simulink model "Masse_MultirotorSimHinf"  (R2018b)
settings: Solver=VariableStepAuto  StartTime=0.0  StopTime=Simulation.T_END  MaxStep=Simulation.TS_MAX  RelTol=1e-3  EnableMultiTasking=on
PreLoadFcn:
  | % InitializeParameters;
undefined symbols (not defined in the file): Aero, armed, ctrl_state, INIT_PARAM_VECTOR, Initial, K_i, K_p, Motor, mpc_att_sp, mpc_ctrl_state, mpc_manual, mpc_pos_sp_triplet, mpc_vehicle_land_detected, mpc_vehicle_status, Simulation, SOF1, SOF2, Uav, Upsilon, v_att_sp, v_control_mode
libraries: simulink_extras x9, simulink x6, dspstat3 x1, Px4Library x1
(part 2 of 11)

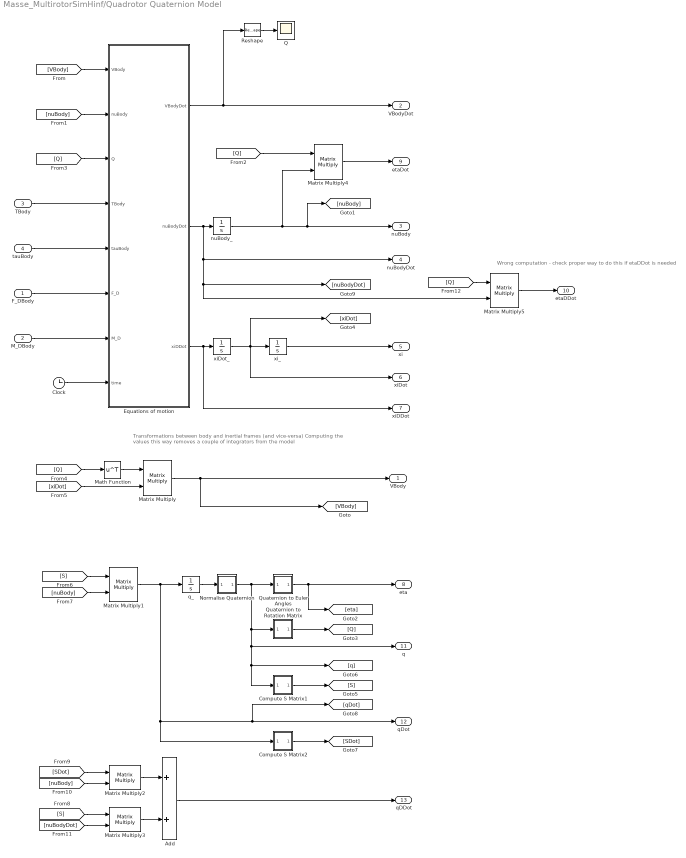
== system Masse_MultirotorSimHinf/Quadrotor Quaternion Model ==
  note: Wrong computation - check proper way to do this if etaDDot is needed
  note: Transformations between body and inertial frames (and vice-versa)
      | Computing the values this way removes a couple of integrators from the model
  F_DBody : Inport  Unit=N
  M_DBody : Inport  Port=2  Unit=N*m
  TBody : Inport  Port=3  Unit=N
  tauBody : Inport  Port=4  Unit=N*m
  Add : Sum
  Clock : Clock
  Compute S Matrix1 : Subsystem  AncestorBlock=QuaternionLibrary/Compute S Matrix
      mask help: Convert an orientation quaternion to an orthogonal transformation matrix
      mask Help:
      | Convert a quaternion
      | [q1 q2 q3 q4]
      | to the S matrix used to compute angular acceleration and velocity quaternion
      | qDot = S * nuBody
      | 
      | qDDot = SDot * nuBody + S * nuBodyDot
      mask Display: disp('S')
  Compute S Matrix2 : Subsystem  AncestorBlock=QuaternionLibrary/Compute S Matrix
      mask help: Convert an orientation quaternion to an orthogonal transformation matrix
      mask Help:
      | Convert a quaternion
      | [q1 q2 q3 q4]
      | to the S matrix used to compute angular acceleration and velocity quaternion
      | qDot = S * nuBody
      | 
      | qDDot = SDot * nuBody + S * nuBodyDot
      mask Display: disp('S')
  Equations of motion : MATLAB Function  TreatAsAtomicUnit=on
  Math Function : Math  Operator=transpose  SaturateOnIntegerOverflow=on
  Matrix Multiply{,1..5} (6 alike) : Product  Multiplication=Matrix(*)
  Normalise Quaternion : Subsystem  AncestorBlock=QuaternionLibrary/Normalise Quaternion
      mask help:
      | Normalise a quaternion
      |
      | Qhat = Q / |Q|
      mask Display: disp('Q/|Q|')
  Q : Scope
  Quaternion to Euler Angles : Subsystem  AncestorBlock=QuaternionLibrary/Quaternion to Euler Angles
      mask help: Convert an orientation quaternion to a vector of Euler angles
      mask Help:
      | Convert an orientation quaternion
      | [q1 q2 q3 q4]
      | where:
      | - q1 is the rotation in radians
      | - [q2 q3 q4] is the vector around which the rotation is performed)
      | to a vector of Euler angles
      | [roll, pitch, yaw]
      | Based on code from the PX4 firmware: https://github.com/PX4/Firmware
      mask Display: disp('Q2E')
  Quaternion to Rotation Matrix : Subsystem  AncestorBlock=QuaternionLibrary/Quaternion to Rotation Matrix
      mask help: Convert an orientation quaternion to an orthogonal transformation matrix
      mask Help:
      | Convert an orientation quaternion
      | [q1 q2 q3 q4]
      | where:
      | - q1 is the rotation in radians
      | - [q2 q3 q4] is the vector around which the rotation is performed)
      | to an orthogonal transformation matrix
      | Based on code from the PX4 firmware: https://github.com/PX4/Firmware
      mask Display: disp('Q2R')
  Reshape : Reshape  OutputDimensionality=Column vector (2-D)
  nuBody_ : Integrator  InitialCondition=Initial.NU_BODY
  q_ : Integrator  InitialCondition=Initial.Q
  xiDot_ : Integrator  InitialCondition=Initial.XI_DOT
  xi_ : Integrator  InitialCondition=Initial.XI
  VBody : Outport  Unit=m/s
  VBodyDot : Outport  Port=2  Unit=m/s^2
  nuBody : Outport  Port=3  Unit=rad/s
  nuBodyDot : Outport  Port=4  Unit=rad/s^2
  xi : Outport  Port=5  Unit=m
  xiDot : Outport  Port=6  Unit=m/s
  xiDDot : Outport  Port=7  Unit=m/s^2
  eta : Outport  Port=8  Unit=rad
  etaDot : Outport  Port=9  Unit=rad/s
  etaDDot : Outport  Port=10  Unit=rad/s^2
  q : Outport  Port=11
  qDot : Outport  Port=12
  qDDot : Outport  Port=13
  wires:
  Equations of motion/1(VBodyDot) -> Reshape/1, VBodyDot/1
  xi_/1 -> xi/1
  [nuBody] -> Equations of motion/2(nuBody)
  [VBody] -> Equations of motion/1(VBody)
  tauBody/1 -> Equations of motion/5(tauBody)
  TBody/1 -> Equations of motion/4(TBody)
  Equations of motion/3(xiDDot) -> xiDot_/1, xiDDot/1
  F_DBody/1 -> Equations of motion/6(F_D)
  Matrix Multiply/1 -> VBody/1, [VBody]
  M_DBody/1 -> Equations of motion/7(M_D)
  nuBody_/1 -> Matrix Multiply4/2, [nuBody], nuBody/1
  Equations of motion/2(nuBodyDot) -> nuBody_/1, nuBodyDot/1, Matrix Multiply5/2, [nuBodyDot]
  q_/1 -> Normalise Quaternion/1(quaternion)
  Quaternion to Euler Angles/1(euler) -> eta/1, [eta]
  Matrix Multiply4/1 -> etaDot/1
  Quaternion to Rotation Matrix/1(rotationMatrix) -> [Q]
  [Q] -> Equations of motion/3(Q)
  [Q] -> Math Function/1
  [xiDot] -> Matrix Multiply/2
  Math Function/1 -> Matrix Multiply/1
  [S] -> Matrix Multiply1/1
  [nuBody] -> Matrix Multiply1/2
  Compute S Matrix2/1(rotationMatrix) -> [SDot]
  [S] -> Matrix Multiply3/1
  Matrix Multiply1/1 -> qDot/1, [qDot], Compute S Matrix2/1(quaternion), q_/1
  [SDot] -> Matrix Multiply2/1
  [nuBody] -> Matrix Multiply2/2
  [nuBodyDot] -> Matrix Multiply3/2
  Matrix Multiply2/1 -> Add/1
  Matrix Multiply3/1 -> Add/2
  Normalise Quaternion/1(normalised) -> Quaternion to Euler Angles/1(quaternion), q/1, Compute S Matrix1/1(quaternion), [q], Quaternion to Rotation Matrix/1(quaternion)
  Compute S Matrix1/1(rotationMatrix) -> [S]
  [Q] -> Matrix Multiply4/1
  Add/1 -> qDDot/1
  [Q] -> Matrix Multiply5/1
  Matrix Multiply5/1 -> etaDDot/1
  Reshape/1 -> Q/1
  xiDot_/1 -> xi_/1, [xiDot], xiDot/1
  Clock/1 -> Equations of motion/8(time)

== system Masse_MultirotorSimHinf/Quaternion to Euler Angles ==
  quaternion : Inport
  MATLAB Function : MATLAB Function  TreatAsAtomicUnit=on
  euler : Outport
  wires:
  quaternion/1 -> MATLAB Function/1(quat)
  MATLAB Function/1(eul) -> euler/1

== system Masse_MultirotorSimHinf/Quaternion to Euler Angles1 ==
  quaternion : Inport
  MATLAB Function : MATLAB Function  TreatAsAtomicUnit=on
  euler : Outport
  wires:
  quaternion/1 -> MATLAB Function/1(quat)
  MATLAB Function/1(eul) -> euler/1

== system Masse_MultirotorSimHinf/SOF1 ==
  y1 : Inport
  Demux : Demux
  Demux1 : Demux  Outputs=2
  Demux2 : Demux  Outputs=2
  Ground : Ground
  Ground1 : Ground
  Manual Switch : ManualSwitch  CurrentSetting=0
  Mux : Mux
  Mux1 : Mux  Inputs=2
  Mux2 : Mux  Inputs=2
  Revert sign : Gain  Gain=-1
  Revert sign1 : Gain  Gain=-1
  SOF1 : Gain  Gain=SOF1  Multiplication=Matrix(K*u)
  SOF1_21-32 : Gain  Gain=-0.76671643026053
  SOF1_23-34 : Gain  Gain=-1.44072900590537
  Sum : Sum  Inputs=+|+
  Sum1 : Sum  Inputs=+|+
  u1 : Outport
  wires:
  Mux/1 -> Manual Switch/2
  Demux/4 -> Mux2/2  "x"
  Demux/3 -> Mux2/1  "y"
  Demux/2 -> Mux1/2  "xdot"
  Demux/1 -> Mux1/1  "ydot"
  Sum1/1 -> Mux/3
  Sum/1 -> Mux/2
  Demux1/1 -> Revert sign/1
  SOF1/1 -> Manual Switch/1
  Manual Switch/1 -> u1/1
  y1/1 -> SOF1/1, Demux/1
  Ground/1 -> Mux/4
  Ground1/1 -> Mux/1
  Demux2/1 -> Revert sign1/1
  SOF1_21-32/1 -> Demux1/1
  Mux1/1 -> SOF1_21-32/1
  Demux1/2 -> Sum1/1
  Mux2/1 -> SOF1_23-34/1
  SOF1_23-34/1 -> Demux2/1
  Demux2/2 -> Sum1/2
  Revert sign/1 -> Sum/1
  Revert sign1/1 -> Sum/2

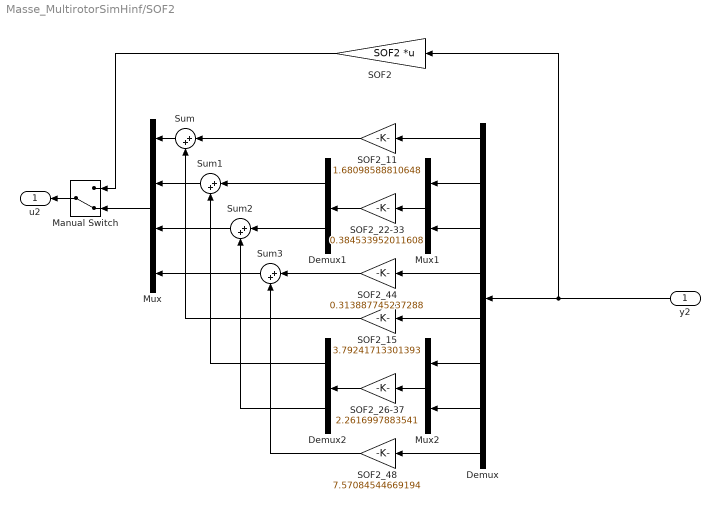
== system Masse_MultirotorSimHinf/SOF2 ==
  y2 : Inport
  Demux : Demux  Outputs=8
  Demux1 : Demux  Outputs=2
  Demux2 : Demux  Outputs=2
  Manual Switch : ManualSwitch  CurrentSetting=0
  Mux : Mux
  Mux1 : Mux  Inputs=2
  Mux2 : Mux  Inputs=2
  SOF2 : Gain  Gain=SOF2  Multiplication=Matrix(K*u)
  SOF2_11 : Gain  Gain=1.68098588810648
  SOF2_15 : Gain  Gain=3.79241713301393
  SOF2_22-33 : Gain  Gain=0.384533952011608
  SOF2_26-37 : Gain  Gain=2.2616997883541
  SOF2_44 : Gain  Gain=0.313887745237288
  SOF2_48 : Gain  Gain=7.57084544669194
  Sum{,1..3} (4 alike) : Sum  Inputs=|++
  u2 : Outport
  wires:
  y2/1 -> SOF2/1, Demux/1
  Manual Switch/1 -> u2/1
  SOF2/1 -> Manual Switch/1
  SOF2_11/1 -> Sum/1
  Demux1/1 -> Sum1/1
  Demux1/2 -> Sum2/1
  SOF2_44/1 -> Sum3/1
  SOF2_15/1 -> Sum/2
  Demux2/1 -> Sum1/2
  Demux2/2 -> Sum2/2
  SOF2_48/1 -> Sum3/2
  Demux/1 -> SOF2_11/1
  Demux/2 -> Mux1/1
  Demux/3 -> Mux1/2
  Demux/4 -> SOF2_44/1
  Demux/5 -> SOF2_15/1
  Demux/6 -> Mux2/1
  Demux/7 -> Mux2/2
  Demux/8 -> SOF2_48/1
  Mux/1 -> Manual Switch/2
  Sum3/1 -> Mux/4
  Sum2/1 -> Mux/3
  Sum1/1 -> Mux/2
  Sum/1 -> Mux/1
  Mux2/1 -> SOF2_26-37/1
  SOF2_26-37/1 -> Demux2/1
  SOF2_22-33/1 -> Demux1/1
  Mux1/1 -> SOF2_22-33/1

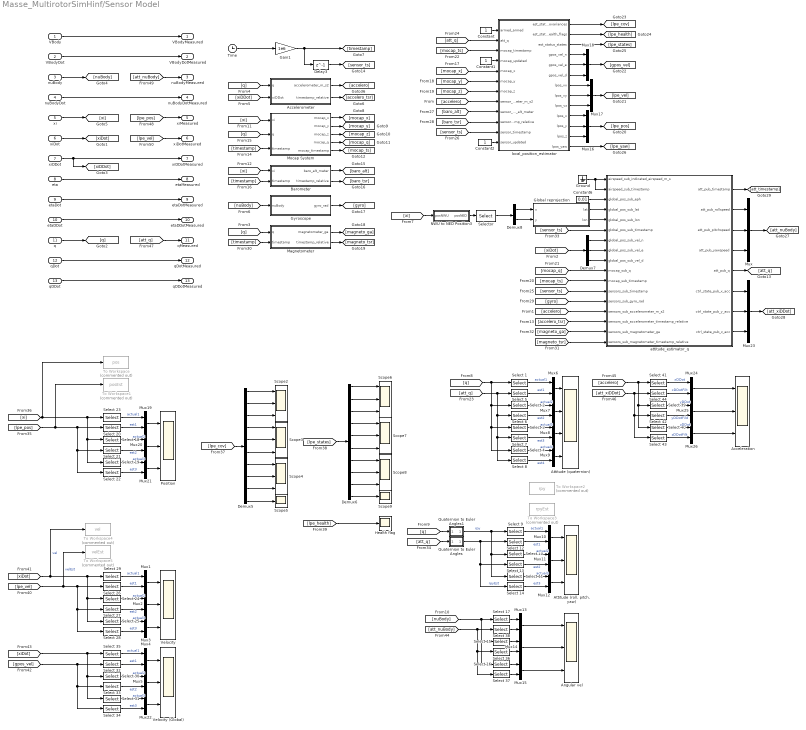
== system Masse_MultirotorSimHinf/Sensor Model ==
  VBody : Inport  Unit=m/s  PortDimensions=3
  VBodyDot : Inport  Port=2  Unit=m/s^2  PortDimensions=3
  nuBody : Inport  Port=3  Unit=rad/s  PortDimensions=3
  nuBodyDot : Inport  Port=4  Unit=rad/s^2  PortDimensions=3
  xi : Inport  Port=5  Unit=m  PortDimensions=3
  xiDot : Inport  Port=6  Unit=m/s  PortDimensions=3
  xiDDot : Inport  Port=7  Unit=m/s^2  PortDimensions=3
  eta : Inport  Port=8  Unit=rad  PortDimensions=3
  etaDot : Inport  Port=9  Unit=rad/s  PortDimensions=3
  etaDDot : Inport  Port=10  Unit=rad/s^2  PortDimensions=3
  q : Inport  Port=11  PortDimensions=4
  qDot : Inport  Port=12  PortDimensions=4
  qDDot : Inport  Port=13  PortDimensions=4
  Acceleration : Scope  NumInputPorts=3
  Accelerometer : Subsystem
  Angular vel : Scope  NumInputPorts=3
  Attitude (quaternion) : Scope  NumInputPorts=4
  "Attitude (roll, pitch, yaw)" : Scope  NumInputPorts=3
  Barometer : Subsystem
  Constant : Constant
  Constant1 : Constant
  Constant2 : Constant
  Constant6 : Constant  Value=0.01
  Delay3 : Delay  DelayLength=1  SampleTime=1/400
  Demux5 : Demux  Outputs=10
  Demux6 : Demux  Outputs=10
  Demux7 : Demux  Outputs=3
  Demux8 : Demux  Outputs=2
  Gain1 : Gain  Gain=1e6
  Global reprojection : Subsystem  AncestorBlock=Px4Library/Global reprojection  mask{LAT0=-36.865577, LON0=174.772065}
      mask prompts: LAT0 "Latitude at [x,y] = [0,0]"; LON0 "Longitude at [x,y] = [0,0]"
      mask Display:
      | disp('REPROJECT')
      | port_label('input', 1, sprintf('x'))
      | port_label('input', 2, sprintf('y'))
      | port_label('output', 1, sprintf('lat'))
      | port_label('output', 2, sprintf('lon'))
  Ground : Ground
  Gyroscope : Subsystem
  Health flag : Scope
  Magnetometer : Subsystem
  Mocap System : Subsystem
  Mux{,16..18,23} (5 alike) : Mux  Inputs=3
  Mux{1..15,19..22,24..26} (22 alike) : Mux  Inputs=2
  NWU to NED Position3 : Subsystem  AncestorBlock=Px4Library/NWU to NED Position  mask(Coordinate transform){}
      mask help:
      | Convert a 3x1 vector or 4x1 quaternion from a North West Up to a North East Down coordinate system.
      |
      | The appropriate coordinate transform is automatically selected based on the input size.
  Position : Scope  NumInputPorts=3
  Quaternion to Euler Angles : Subsystem  AncestorBlock=QuaternionLibrary/Quaternion to Euler Angles
      mask help: Convert an orientation quaternion to a vector of Euler angles
      mask Help:
      | Convert an orientation quaternion
      | [q1 q2 q3 q4]
      | where:
      | - q1 is the rotation in radians
      | - [q2 q3 q4] is the vector around which the rotation is performed)
      | to a vector of Euler angles
      | [roll, pitch, yaw]
      | Based on code from the PX4 firmware: https://github.com/PX4/Firmware
      mask Display: disp('Q2E')
  Quaternion to Euler Angles1 : Subsystem  AncestorBlock=QuaternionLibrary/Quaternion to Euler Angles
      mask help: Convert an orientation quaternion to a vector of Euler angles
      mask Help:
      | Convert an orientation quaternion
      | [q1 q2 q3 q4]
      | where:
      | - q1 is the rotation in radians
      | - [q2 q3 q4] is the vector around which the rotation is performed)
      | to a vector of Euler angles
      | [roll, pitch, yaw]
      | Based on code from the PX4 firmware: https://github.com/PX4/Firmware
      mask Display: disp('Q2E')
  Scope{2..4,6..8} (6 alike) : Scope  NumInputPorts=3
  Scope5 : Scope
  Scope9 : Scope
  Select 1 : Selector  InputPortWidth=4  IndexOptions=Index vector (dialog)  Indices=1  OutputSizes=1
  Select {10,13,15,18,21,24,27,30,33,36,39,42} (12 alike) : Selector  InputPortWidth=3  IndexOptions=Index vector (dialog)  Indices=2  OutputSizes=1
  Select {11,14,16,19,22,25,28,31,34,37,40,43} (12 alike) : Selector  InputPortWidth=3  IndexOptions=Index vector (dialog)  Indices=3  OutputSizes=1
  Select {9,12,17,20,23,26,29,32,35,38,41,44} (12 alike) : Selector  InputPortWidth=3  IndexOptions=Index vector (dialog)  Indices=1  OutputSizes=1
  Select 2 : Selector  InputPortWidth=4  IndexOptions=Index vector (dialog)  Indices=2  OutputSizes=1
  Select 3 : Selector  InputPortWidth=4  IndexOptions=Index vector (dialog)  Indices=3  OutputSizes=1
  Select 4 : Selector  InputPortWidth=4  IndexOptions=Index vector (dialog)  Indices=4  OutputSizes=1
  Select 5 : Selector  InputPortWidth=4  IndexOptions=Index vector (dialog)  Indices=1  OutputSizes=1
  Select 6 : Selector  InputPortWidth=4  IndexOptions=Index vector (dialog)  Indices=2  OutputSizes=1
  Select 7 : Selector  InputPortWidth=4  IndexOptions=Index vector (dialog)  Indices=3  OutputSizes=1
  Select 8 : Selector  InputPortWidth=4  IndexOptions=Index vector (dialog)  Indices=4  OutputSizes=1
  Selector : Selector  InputPortWidth=3  IndexOptions=Index vector (dialog)  Indices=[1 2]  OutputSizes=1
  Time : Clock
  To Workspace : ToWorkspace  Commented=on  VariableName=pos  SaveFormat=Structure With Time  SampleTime=-1
  To Workspace1 : ToWorkspace  Commented=on  VariableName=posEst  SaveFormat=Structure With Time  SampleTime=-1
  To Workspace2 : ToWorkspace  Commented=on  VariableName=rpy  SaveFormat=Structure With Time  SampleTime=-1
  To Workspace3 : ToWorkspace  Commented=on  VariableName=rpyEst  SaveFormat=Structure With Time  SampleTime=-1
  To Workspace4 : ToWorkspace  Commented=on  VariableName=vel  SaveFormat=Structure With Time  SampleTime=-1
  To Workspace5 : ToWorkspace  Commented=on  VariableName=velEst  SaveFormat=Structure With Time  SampleTime=-1
  Velocity : Scope  NumInputPorts=3
  Velocity (Global) : Scope  NumInputPorts=3
  attitude_estimator_q : Subsystem  AncestorBlock=Px4Library/attitude_estimator_q  mask(PX4 LPE (local position estimator): local_position_estimator){Q_SAMPLING_PERIOD=1/250, INIT_Q=[0.99812 -1.4569e-22   -0.061217 -8.9353e-24], ATT_W_ACC=0.2, ATT_W_MAG=0.1, ATT_W_EXT_HDG=0.1, ATT_W_GYRO_BIAS=0.1, ATT_MAG_DECL=0, ATT_MAG_DECL_A=1, ATT_EXT_HDG_M=2, ATT_ACC_COMP=1, ATT_BIAS_MAX=0.05, FW_ARSP_MODE=0}
      mask prompts: Q_SAMPLING_PERIOD "Sampling period (s)"; INIT_Q "INIT_Q - Initial UAV orientation - set to 0 to let controller decide (bugged) (-)"; ATT_W_ACC "ATT_W_ACC - Complimentary filter accelerometer weight (-)"; ATT_W_MAG "ATT_W_MAG - Complimentary filter magnetometer weight (-)"; ATT_W_EXT_HDG "ATT_W_EXT_HDG - Complimentary filter external heading weight (-)"; ATT_W_GYRO_BIAS "ATT_W_GYRO_BIAS - Complimentary filter gyroscope bias weight (-)"; ATT_MAG_DECL "ATT_MAG_DECL - Magnetic declination. Not used when GPS available (deg)"; ATT_MAG_DECL_A "ATT_MAG_DECL_A - Automatic GPS based declination compensation (-)"; ATT_EXT_HDG_M "ATT_EXT_HDG_M - External heading usage mode (from Motion capture/Vision) (-), 0 None 1 Vision 2 Motion Capture"; ATT_ACC_COMP "ATT_ACC_COMP - Acceleration compensation based on GPS velocity. (-)"; ATT_BIAS_MAX "ATT_BIAS_MAX - Gyro bias limit (rad/s)"; FW_ARSP_MODE "FW_ARSP_MODE - Method used to publish the airspeed (-), 0 Measured airspeed 1 Vehicle ground speed 2 Airspeed invalid"
      mask TypeOptions ATT_EXT_HDG_M: 0 | 1 | 2
      mask TypeOptions FW_ARSP_MODE: 0 | 1 | 2
  local_position_estimator : Subsystem  AncestorBlock=Px4Library/local_position_estimator  mask(PX4 LPE (local position estimator): local_position_estimator){LPE_SAMPLING_PERIOD=0.01, LPE_ACC_XY=0.012, LPE_ACC_Z=0.02, LPE_BAR_Z=3, LPE_EPH_MAX=3, LPE_EPV_MAX=5, LPE_FAKE_ORIGIN=0, LPE_FGYRO_HP=0.001, LPE_FLW_OFF_Z=0, LPE_FLW_QMIN=150, LPE_FLW_R=7, LPE_FLW_RR=7, LPE_FLW_SCALE=1.3, LPE_GPS_DELAY=0.29, LPE_GPS_VXY=0.25, LPE_GPS_VZ=0.25, LPE_GPS_XY=1, LPE_GPS_Z=3, LPE_LAND_VXY=0.05, LPE_LAND_Z=0.03, LPE_LAT=40.43, LPE_LDR_OFF_Z=0, LPE_LDR_Z=0.03, LPE_LON=-86.929, LPE_PN_B=0.001, LPE_PN_P=0.1, LPE_PN_T=0.001, LPE_PN_V=0.1, LPE_SNR_OFF_Z=0, LPE_SNR_Z=0.05, LPE_T_MAX_GRADE=1, LPE_VIC_P=0.001, LPE_VIS_DELAY=0.1, LPE_VIS_XY=0.1, LPE_VIS_Z=0.5, LPE_VXY_PUB=0.3, LPE_X_LP=5, LPE_Z_PUB=1, LPE_FUSION=193, Barometer=on, GPS=off, LIDAR=off, Flow=off, Sonar=off, Vision=off, Mocap=on, Land=on}
      mask prompts: LPE_SAMPLING_PERIOD "Sampling period (s)"; LPE_ACC_XY "LPE_ACC_XY - Accelerometer xy noise density (m/s^2/sqrt(Hz))"; LPE_ACC_Z "LPE_ACC_Z - Accelerometer z noise density (m/s^2/sqrt(Hz))"; LPE_BAR_Z "LPE_BAR_Z - Barometric presssure altitude z standard deviation. (m)"; LPE_EPH_MAX "LPE_EPH_MAX - Max EPH allowed for GPS initialization (m)"; LPE_EPV_MAX "LPE_EPV_MAX - Max EPV allowed for GPS initialization (m)"; LPE_FAKE_ORIGIN "LPE_FAKE_ORIGIN - Enable publishing of a fake global position (e.g for AUTO missions using Optical Flow) (-)"; LPE_FGYRO_HP "LPE_FGYRO_HP - Flow gyro high pass filter cut off frequency (Hz)"; LPE_FLW_OFF_Z "LPE_FLW_OFF_Z - Optical flow z offset from center (m)"; LPE_FLW_QMIN "LPE_FLW_QMIN - Optical flow minimum quality threshold (-)"; LPE_FLW_R "LPE_FLW_R - Optical flow rotation (roll/pitch) noise gain (m/s / (rad))"; LPE_FLW_RR "LPE_FLW_RR - Optical flow angular velocity noise gain (m/s / (rad/s))"; LPE_FLW_SCALE "LPE_FLW_SCALE - Optical flow scale (m)"; LPE_GPS_DELAY "LPE_GPS_DELAY - GPS delay compensaton (sec)"; LPE_GPS_VXY "LPE_GPS_VXY - GPS xy velocity standard deviation. (m/s)"; LPE_GPS_VZ "LPE_GPS_VZ - GPS z velocity standard deviation. (m/s)"; LPE_GPS_XY "LPE_GPS_XY - Minimum GPS xy standard deviation, uses reported EPH if greater. (m)"; LPE_GPS_Z "LPE_GPS_Z - Minimum GPS z standard deviation, uses reported EPV if greater. (m)"; LPE_LAND_VXY "LPE_LAND_VXY - Land detector xy velocity standard deviation (m/s)"; LPE_LAND_Z "LPE_LAND_Z - Land detector z standard deviation (m)"; LPE_LAT "LPE_LAT - Local origin latitude for nav w/o GPS (deg)"; LPE_LDR_OFF_Z "LPE_LDR_OFF_Z - Lidar z offset from center of vehicle +down (m)"; LPE_LDR_Z "LPE_LDR_Z - Lidar z standard deviation. (m)"; LPE_LON "LPE_LON - Local origin longitude for nav w/o GPS (deg)"; LPE_PN_B "LPE_PN_B - Accel bias propagation noise density ((m/s^2)/s/sqrt(Hz))"; LPE_PN_P "LPE_PN_P - Position propagation noise density (m/s/sqrt(Hz))"; LPE_PN_T "LPE_PN_T - Terrain random walk noise density, hilly/outdoor (0.1), flat/Indoor (0.001) ((m/s)/(sqrt(hz)))"; LPE_PN_V "LPE_PN_V - Velocity propagation noise density ((m/s)/s/sqrt(Hz))"; LPE_SNR_OFF_Z "LPE_SNR_OFF_Z - Sonar z offset from center of vehicle +down (m)"; LPE_SNR_Z "LPE_SNR_Z - Sonar z standard deviation. (m)"; LPE_T_MAX_GRADE "LPE_T_MAX_GRADE - Terrain maximum percent grade, hilly/outdoor (100 = 45 deg), flat/Indoor (0 = 0 deg) (%)"; LPE_VIC_P "LPE_VIC_P - Vicon position standard deviation. (m)"; LPE_VIS_DELAY "LPE_VIS_DELAY - Vision delay compensaton. (sec)"; LPE_VIS_XY "LPE_VIS_XY - Vision xy standard deviation. (m)"; LPE_VIS_Z "LPE_VIS_Z - Vision z standard deviation. (m)"; LPE_VXY_PUB "LPE_VXY_PUB - Required velocity xy standard deviation to publish position (m/s)"; LPE_X_LP "LPE_X_LP - Cut frequency for state publication (Hz)"; LPE_Z_PUB "LPE_Z_PUB - Required z standard deviation to publish altitude/ terrain (m)"; LPE_FUSION "LPE_FUSION - Integer bitmask controlling data fusion (-)"; Barometer "Use Barometer"; GPS "Use GPS"; LIDAR "Use LIDAR"; Flow "Use Flow"; Sonar "Use Sonar"; Vision "Use Vision"; Mocap "Use Mocap"; Land "Use Land"
      mask Callback Barometer:
      | status = get_param( gcb, 'Barometer' );
      | if strcmp( status, 'on' )
      | 	lpe = bitor( uint8(str2num(get_param( gcb, 'LPE_FUSION' ))), uint8(2^0) );
      | 	set_param( gcb, 'LPE_FUSION', num2str(lpe) );
      | else
      | 	lpe = bitand( uint8(str2num(get_param( gcb, 'LPE_FUSION' ))), bitcmp(uint8(2^0), 'uint8' ));
      | 	set_param( gcb, 'LPE_FUSION', num2str(lpe) );
      | end
      mask Callback GPS:
      | status = get_param( gcb, 'GPS' );
      | if strcmp( status, 'on' )
      | 	lpe = bitor( uint8(str2num(get_param( gcb, 'LPE_FUSION' ))), uint8(2^1) );
      | 	set_param( gcb, 'LPE_FUSION', num2str(lpe) );
      | else
      | 	lpe = bitand( uint8(str2num(get_param( gcb, 'LPE_FUSION' ))), bitcmp(uint8(2^1), 'uint8' ));
      | 	set_param( gcb, 'LPE_FUSION', num2str(lpe) );
      | end
      mask Callback LIDAR:
      | status = get_param( gcb, 'LIDAR' );
      | if strcmp( status, 'on' )
      | 	lpe = bitor( uint8(str2num(get_param( gcb, 'LPE_FUSION' ))), uint8(2^2) );
      | 	set_param( gcb, 'LPE_FUSION', num2str(lpe) );
      | else
      | 	lpe = bitand( uint8(str2num(get_param( gcb, 'LPE_FUSION' ))), bitcmp(uint8(2^2), 'uint8' ));
      | 	set_param( gcb, 'LPE_FUSION', num2str(lpe) );
      | end
      mask Callback Flow:
      | status = get_param( gcb, 'Flow' );
      | if strcmp( status, 'on' )
      | 	lpe = bitor( uint8(str2num(get_param( gcb, 'LPE_FUSION' ))), uint8(2^3) );
      | 	set_param( gcb, 'LPE_FUSION', num2str(lpe) );
      | else
      | 	lpe = bitand( uint8(str2num(get_param( gcb, 'LPE_FUSION' ))), bitcmp(uint8(2^3), 'uint8' ));
      | 	set_param( gcb, 'LPE_FUSION', num2str(lpe) );
      | end
      mask Callback Sonar:
      | status = get_param( gcb, 'Sonar' );
      | if strcmp( status, 'on' )
      | 	lpe = bitor( uint8(str2num(get_param( gcb, 'LPE_FUSION' ))), uint8(2^4) );
      | 	set_param( gcb, 'LPE_FUSION', num2str(lpe) );
      | else
      | 	lpe = bitand( uint8(str2num(get_param( gcb, 'LPE_FUSION' ))), bitcmp(uint8(2^4), 'uint8' ));
      | 	set_param( gcb, 'LPE_FUSION', num2str(lpe) );
      | end
      mask Callback Vision:
      | status = get_param( gcb, 'Vision' );
      | if strcmp( status, 'on' )
      | 	lpe = bitor( uint8(str2num(get_param( gcb, 'LPE_FUSION' ))), uint8(2^5) );
      | 	set_param( gcb, 'LPE_FUSION', num2str(lpe) );
      | else
      | 	lpe = bitand( uint8(str2num(get_param( gcb, 'LPE_FUSION' ))), bitcmp(uint8(2^5), 'uint8' ));
      | 	set_param( gcb, 'LPE_FUSION', num2str(lpe) );
      | end
      mask Callback Mocap:
      | status = get_param( gcb, 'Mocap' );
      | if strcmp( status, 'on' )
      | 	lpe = bitor( uint8(str2num(get_param( gcb, 'LPE_FUSION' ))), uint8(2^6) );
      | 	set_param( gcb, 'LPE_FUSION', num2str(lpe) );
      | else
      | 	lpe = bitand( uint8(str2num(get_param( gcb, 'LPE_FUSION' ))), bitcmp(uint8(2^6), 'uint8' ));
      | 	set_param( gcb, 'LPE_FUSION', num2str(lpe) );
      | end
      mask Callback Land:
      | status = get_param( gcb, 'Land' );
      | if strcmp( status, 'on' )
      | 	lpe = bitor( uint8(str2num(get_param( gcb, 'LPE_FUSION' ))), uint8(2^7) );
      | 	set_param( gcb, 'LPE_FUSION', num2str(lpe) );
      | else
      | 	lpe = bitand( uint8(str2num(get_param( gcb, 'LPE_FUSION' ))), bitcmp(uint8(2^7), 'uint8' ));
      | 	set_param( gcb, 'LPE_FUSION', num2str(lpe) );
      | end
  VBodyMeasured : Outport  Unit=m/s
  VBodyDotMeasured : Outport  Port=2  Unit=m/s^2
  nuBodyMeasured : Outport  Port=3  Unit=rad/s
  nuBodyDotMeasured : Outport  Port=4  Unit=rad/s^2
  xiMeasured : Outport  Port=5  Unit=m
  xiDotMeasured : Outport  Port=6  Unit=m/s
  xiDDotMeasured : Outport  Port=7  Unit=m/s^2
  etaMeasured : Outport  Port=8  Unit=rad
  etaDotMeasured : Outport  Port=9  Unit=rad/s
  etaDDotMeasured : Outport  Port=10  Unit=rad/s^2
  qMeasured : Outport  Port=11
  qDotMeasured : Outport  Port=12
  qDDotMeasured : Outport  Port=13
  wires:
  xiDot/1 -> [xiDot]
  xi/1 -> [xi]
  nuBodyDot/1 -> nuBodyDotMeasured/1
  nuBody/1 -> [nuBody]
  VBodyDot/1 -> VBodyDotMeasured/1
  VBody/1 -> VBodyMeasured/1
  eta/1 -> etaMeasured/1
  etaDot/1 -> etaDotMeasured/1
  etaDDot/1 -> etaDDotMeasured/1
  q/1 -> [q]
  qDot/1 -> qDotMeasured/1
  qDDot/1 -> qDDotMeasured/1
  [att_q] -> local_position_estimator/2(att_q)
  [mocap_x] -> local_position_estimator/5(mocap_x)
  [mocap_z] -> local_position_estimator/7(mocap_z)
  local_position_estimator/10(lpos_x) -> Mux16/1
  local_position_estimator/11(lpos_y) -> Mux16/2
  local_position_estimator/12(lpos_z) -> Mux16/3
  Demux5/2 -> Scope2/2
  Demux5/1 -> Scope2/1
  Demux5/3 -> Scope2/3
  Demux5/4 -> Scope3/1
  Demux5/5 -> Scope3/2
  Demux5/6 -> Scope3/3
  Demux5/7 -> Scope4/1
  Demux5/8 -> Scope4/2
  Demux5/9 -> Scope4/3
  Demux5/10 -> Scope5/1
  [lpe_states] -> Demux6/1
  Demux6/2 -> Scope6/2
  Demux6/1 -> Scope6/1
  Demux6/3 -> Scope6/3
  Demux6/4 -> Scope7/1
  Demux6/5 -> Scope7/2
  Demux6/6 -> Scope7/3
  Demux6/7 -> Scope8/1
  Demux6/8 -> Scope8/2
  Demux6/9 -> Scope8/3
  Demux6/10 -> Scope9/1
  Constant1/1 -> local_position_estimator/4(mocap_updated)
  [lpe_health] -> Health flag/1
  Constant/1 -> local_position_estimator/1(armed_armed)
  [mocap_ts] -> local_position_estimator/3(mocap_timestamp)
  [xiDot] -> Demux7/1
  Time/1 -> Gain1/1
  [accelero_tsr] -> attitude_estimator_q/15(sensors_sub_accelerometer_timestamp_relative)
  Global reprojection/1(lat) -> attitude_estimator_q/4(global_pos_sub_lat)
  Global reprojection/2(lon) -> attitude_estimator_q/5(global_pos_sub_lon)
  [xi] -> NWU to NED Position3/1(posNWU)
  NWU to NED Position3/1(posNED) -> Selector/1
  Selector/1 -> Demux8/1
  Demux8/1 -> Global reprojection/1(x)
  Demux8/2 -> Global reprojection/2(y)
  [att_q] -> Select 8/1, Select 7/1, Select 6/1, Select 5/1
  [q] -> Select 2/1, Select 3/1, Select 4/1, Select 1/1
  Mux6/1 -> Attitude (quaternion)/1
  Mux7/1 -> Attitude (quaternion)/2
  Mux8/1 -> Attitude (quaternion)/3
  Mux9/1 -> Attitude (quaternion)/4
  Select 4/1 -> Mux9/1  "actual4"
  Select 8/1 -> Mux9/2  "est4"
  Select 3/1 -> Mux8/1  "actual3"
  Select 7/1 -> Mux8/2  "est3"
  Select 6/1 -> Mux7/2  "est2"
  Select 2/1 -> Mux7/1  "actual2"
  Select 5/1 -> Mux6/2  "est1"
  Select 1/1 -> Mux6/1  "actual1"
  Constant6/1 -> attitude_estimator_q/3(global_pos_sub_eph)
  [q] -> Magnetometer/1(q)
  Mux10/1 -> "Attitude (roll, pitch, yaw)"/1
  Mux11/1 -> "Attitude (roll, pitch, yaw)"/2
  Mux12/1 -> "Attitude (roll, pitch, yaw)"/3
  Select 11/1 -> Mux12/1  "actual3"
  Select 14/1 -> Mux12/2  "est3"
  Select 13/1 -> Mux11/2  "est2"
  Select 10/1 -> Mux11/1  "actual2"
  Select 12/1 -> Mux10/2  "est1"
  Select 9/1 -> Mux10/1  "actual1"
  [q] -> Quaternion to Euler Angles1/1(quaternion)
  Quaternion to Euler Angles1/1(euler) -> Select 11/1, Select 10/1, Select 9/1  "rpy"
  Quaternion to Euler Angles/1(euler) -> Select 14/1, Select 13/1, Select 12/1  "rpyEst"
  Mux13/1 -> Angular vel/1
  Mux14/1 -> Angular vel/2
  Mux15/1 -> Angular vel/3
  Select 17/1 -> Mux13/1
  Select 15/1 -> Mux14/1
  Select 16/1 -> Mux15/1
  [nuBody] -> Select 17/1, Select 16/1, Select 15/1
  Demux7/2 -> attitude_estimator_q/8(global_pos_sub_vel_e)
  [accelero] -> attitude_estimator_q/14(sensors_sub_accelerometer_m_s2)
  [sensor_ts] -> attitude_estimator_q/12(sensors_sub_timestamp)
  [magneto_ga] -> attitude_estimator_q/16(sensors_sub_magnetometer_ga)
  [nuBody] -> Gyroscope/1(nuBody)
  [gyro] -> attitude_estimator_q/13(sensors_sub_gyro_rad)
  [q] -> Accelerometer/1(q)
  [xiDDot] -> Accelerometer/2(xiDDot)
  Accelerometer/1(accelerometer_m_s2) -> [accelero]
  Accelerometer/2(timestamp_relative) -> [accelero_tsr]
  [mocap_q] -> attitude_estimator_q/10(mocap_sub_q)
  [mocap_ts] -> attitude_estimator_q/11(mocap_sub_timestamp)
  Gain1/1 -> Delay3/1, [timestamp]
  [timestamp] -> Mocap System/3(timestamp)
  [q] -> Mocap System/2(q)
  [xi] -> Mocap System/1(xi)
  Constant2/1 -> local_position_estimator/12(sensor_updated)
  [baro_alt] -> local_position_estimator/9(sensor_baro_alt_meter)
  [baro_tsr] -> local_position_estimator/10(sensor_baro_timestamp_relative)
  Mocap System/1(mocap_x) -> [mocap_x]
  Mocap System/2(mocap_y) -> [mocap_y]
  Mocap System/3(mocap_z) -> [mocap_z]
  [mocap_y] -> local_position_estimator/6(mocap_y)
  Mocap System/4(mocap_q) -> [mocap_q]
  Mocap System/5(mocap_timestamp) -> [mocap_ts]
  attitude_estimator_q/5(att_pub_q) -> [att_q]
  Delay3/1 -> [sensor_ts]
  [sensor_ts] -> local_position_estimator/11(sensor_timestamp)
  [xi] -> Barometer/1(xi)
  [timestamp] -> Barometer/2(timestamp)
  Barometer/1(baro_alt_meter) -> [baro_alt]
  Barometer/2(timestamp_relative) -> [baro_tsr]
  Gyroscope/1(gyro_rad) -> [gyro]
  [timestamp] -> Magnetometer/2(timestamp)
  Magnetometer/2(timestamp_relative) -> [magneto_tsr]
  Magnetometer/1(magnetometer_ga) -> [magneto_ga]
  [magneto_tsr] -> attitude_estimator_q/17(sensors_sub_magnetometer_timestamp_relative)
  Demux7/1 -> attitude_estimator_q/7(global_pos_sub_vel_n)
  Demux7/3 -> attitude_estimator_q/9(global_pos_sub_vel_d)
  [sensor_ts] -> attitude_estimator_q/6(global_pos_sub_timestamp)
  Mux16/1 -> [lpe_pos]
  local_position_estimator/7(lpos_vx) -> Mux17/1
  local_position_estimator/8(lpos_vy) -> Mux17/2
  local_position_estimator/9(lpos_vz) -> Mux17/3
  Mux17/1 -> [lpe_vel]
  local_position_estimator/4(gpos_vel_n) -> Mux18/1
  local_position_estimator/5(gpos_vel_e) -> Mux18/2
  local_position_estimator/6(gpos_vel_d) -> Mux18/3
  Mux18/1 -> [gpos_vel]
  local_position_estimator/1(est_status_covariances) -> [lpe_cov]
  local_position_estimator/2(est_status_health_flags) -> [lpe_health]
  local_position_estimator/3(est_status_states) -> [lpe_states]
  [att_q] -> Quaternion to Euler Angles/1(quaternion)
  Mux19/1 -> Position/1
  Mux20/1 -> Position/2
  Mux21/1 -> Position/3
  Select 19/1 -> Mux21/1  "actual3"
  Select 22/1 -> Mux21/2  "est3"
  Select 21/1 -> Mux20/2  "est2"
  Select 18/1 -> Mux20/1  "actual2"
  Select 20/1 -> Mux19/2  "est1"
  Select 23/1 -> Mux19/1  "actual1"
  [lpe_pos] -> To Workspace1/1, Select 20/1, Select 21/1, Select 22/1
  [lpe_cov] -> Demux5/1
  [xi] -> Select 23/1, Select 18/1, Select 19/1, To Workspace/1
  Mux1/1 -> Velocity/1
  Mux2/1 -> Velocity/2
  Mux3/1 -> Velocity/3
  Select 25/1 -> Mux3/1  "actual3"
  Select 28/1 -> Mux3/2  "est3"
  Select 27/1 -> Mux2/2  "est2"
  Select 24/1 -> Mux2/1  "actual2"
  Select 26/1 -> Mux1/2  "est1"
  Select 29/1 -> Mux1/1  "actual1"
  [lpe_vel] -> To Workspace5/1, Select 28/1, Select 27/1, Select 26/1  "velEst"
  [xiDot] -> To Workspace4/1, Select 25/1, Select 24/1, Select 29/1  "vel"
  Mux4/1 -> Velocity (Global)/1
  Mux5/1 -> Velocity (Global)/2
  Mux22/1 -> Velocity (Global)/3
  Select 31/1 -> Mux22/1  "actual3"
  Select 34/1 -> Mux22/2  "est3"
  Select 33/1 -> Mux5/2  "est2"
  Select 30/1 -> Mux5/1  "actual2"
  Select 32/1 -> Mux4/2  "est1"
  Select 35/1 -> Mux4/1  "actual1"
  [gpos_vel] -> Select 32/1, Select 33/1, Select 34/1
  [xiDot] -> Select 35/1, Select 30/1, Select 31/1
  [accelero] -> local_position_estimator/8(sensor_accelerometer_m_s2)
  local_position_estimator/13(lpos_yaw) -> [lpe_yaw]
  Mux/1 -> [att_nuBody]
  attitude_estimator_q/3(att_pub_pitchspeed) -> Mux/2
  attitude_estimator_q/2(att_pub_rollspeed) -> Mux/1
  attitude_estimator_q/4(att_pub_yawspeed) -> Mux/3
  Select 38/1 -> Mux13/2
  Select 37/1 -> Mux15/2
  [att_nuBody] -> Select 38/1, Select 36/1, Select 37/1
  Select 36/1 -> Mux14/2
  Mux23/1 -> [att_xiDDot]
  attitude_estimator_q/7(ctrl_state_pub_y_acc) -> Mux23/2
  attitude_estimator_q/6(ctrl_state_pub_x_acc) -> Mux23/1
  attitude_estimator_q/8(ctrl_state_pub_z_acc) -> Mux23/3
  Mux24/1 -> Acceleration/1
  Mux25/1 -> Acceleration/2
  Mux26/1 -> Acceleration/3
  Select 41/1 -> Mux24/1  "xDDot"
  Select 39/1 -> Mux25/1  "yDDot"
  Select 40/1 -> Mux26/1  "zDDot"
  [accelero] -> Select 39/1, Select 40/1, Select 41/1
  Select 44/1 -> Mux24/2  "xDDotFilt"
  Select 43/1 -> Mux26/2  "zDDotFilt"
  [att_xiDDot] -> Select 43/1, Select 42/1, Select 44/1
  Select 42/1 -> Mux25/2  "yDDotFild"
  attitude_estimator_q/1(att_pub_timestamp) -> [att_timestamp]
  [att_q] -> qMeasured/1
  [att_nuBody] -> nuBodyMeasured/1
  xiDDot/1 -> xiDDotMeasured/1, [xiDDot]
  [lpe_pos] -> xiMeasured/1
  [lpe_vel] -> xiDotMeasured/1
  Ground/1 -> attitude_estimator_q/2(airspeed_sub_timestamp), attitude_estimator_q/1(airspeed_sub_indicated_airspeed_m_s)

== system Masse_MultirotorSimHinf/Stick logging buffer ==
  stickIn : Inport
  stickOut : Outport
  wires:
  stickIn/1 -> stickOut/1

== system Masse_MultirotorSimHinf/att_NWUtoNED ==
  posNWU : Inport
  Multiply : Product  Inputs=**
  Position gain : Constant  Value=[1; -1; -1]
  posNED : Outport
  wires:
  posNWU/1 -> Multiply/1
  Multiply/1 -> posNED/1
  Position gain/1 -> Multiply/2

== system Masse_MultirotorSimHinf/att_mixerInput ==
  qPosCtrl : Inport
  qInput : Inport  Port=2
  Euler Angles to Quaternion : Subsystem  AncestorBlock=QuaternionLibrary/Euler Angles to Quaternion
      mask help: Convert vector of Euler angles to an orientation quaternion
      mask Help:
      | Convert vector of Euler angles
      | [roll, pitch, yaw]
      | to an orientation quaternion
      | [q1 q2 q3 q4]
      | where:
      | - q1 is the rotation in radians
      | - [q2 q3 q4] is the vector around which the rotation is performed)
      | 
      | Based on code from the PX4 firmware: https://github.com/PX4/Firmware
      mask Display: disp('E2Q')
  Mux : Mux  Inputs=3
  Quaternion to Euler Angles2 : Subsystem  AncestorBlock=QuaternionLibrary/Quaternion to Euler Angles
      mask help: Convert an orientation quaternion to a vector of Euler angles
      mask Help:
      | Convert an orientation quaternion
      | [q1 q2 q3 q4]
      | where:
      | - q1 is the rotation in radians
      | - [q2 q3 q4] is the vector around which the rotation is performed)
      | to a vector of Euler angles
      | [roll, pitch, yaw]
      | Based on code from the PX4 firmware: https://github.com/PX4/Firmware
      mask Display: disp('Q2E')
  Quaternion to Euler Angles3 : Subsystem  AncestorBlock=QuaternionLibrary/Quaternion to Euler Angles
      mask help: Convert an orientation quaternion to a vector of Euler angles
      mask Help:
      | Convert an orientation quaternion
      | [q1 q2 q3 q4]
      | where:
      | - q1 is the rotation in radians
      | - [q2 q3 q4] is the vector around which the rotation is performed)
      | to a vector of Euler angles
      | [roll, pitch, yaw]
      | Based on code from the PX4 firmware: https://github.com/PX4/Firmware
      mask Display: disp('Q2E')
  Selector25 : Selector  InputPortWidth=3  IndexOptions=Index vector (dialog)  Indices=1  OutputSizes=1
  Selector27 : Selector  InputPortWidth=3  IndexOptions=Index vector (dialog)  Indices=3  OutputSizes=1
  Selector28 : Selector  InputPortWidth=3  IndexOptions=Index vector (dialog)  Indices=2  OutputSizes=1
  qDes : Outport
  wires:
  qPosCtrl/1 -> Quaternion to Euler Angles2/1(quaternion)
  qInput/1 -> Quaternion to Euler Angles3/1(quaternion)
  Euler Angles to Quaternion/1(quaternion) -> qDes/1
  Mux/1 -> Euler Angles to Quaternion/1(euler)
  Quaternion to Euler Angles2/1(euler) -> Selector25/1
  Quaternion to Euler Angles3/1(euler) -> Selector27/1, Selector28/1
  Selector25/1 -> Mux/1
  Selector27/1 -> Mux/3
  Selector28/1 -> Mux/2

== system Masse_MultirotorSimHinf/att_q_NWUtoNED ==
  qNWU : Inport
  Multiply : Product  Inputs=**
  Quaternion gain : Constant  Value=[1; 1; -1; -1]
  qNED : Outport
  wires:
  Quaternion gain/1 -> Multiply/2
  Multiply/1 -> qNED/1
  qNWU/1 -> Multiply/1

== system Masse_MultirotorSimHinf/mc_att_control ==
  armed : Inport  PortDimensions=1  SampleTime=MC_SAMPLING_PERIOD
  flags : Inport  Port=2  PortDimensions=5  SampleTime=MC_SAMPLING_PERIOD
  qDes : Inport  Port=3  PortDimensions=4  SampleTime=MC_SAMPLING_PERIOD
  thrustDes : Inport  Port=4  PortDimensions=1  SampleTime=MC_SAMPLING_PERIOD
  yawRateDes : Inport  Port=5  PortDimensions=1  SampleTime=MC_SAMPLING_PERIOD
  q : Inport  Port=6  PortDimensions=4  SampleTime=MC_SAMPLING_PERIOD
  nuBody : Inport  Port=7  PortDimensions=3  SampleTime=MC_SAMPLING_PERIOD
  Bus Selector1 : BusSelector  OutputSignals=actuators.control
  Clock : Clock
  Control inputs : BusAssignment  AssignedSignals=v_att_sp.q_d,v_att_sp.thrust,v_att_sp.yaw_sp_move_rate
  Demux : Demux  Outputs=3
  Demux1 : Demux  Outputs=5
  Feedback inputs : BusAssignment  AssignedSignals=ctrl_state.q,ctrl_state.roll_rate,ctrl_state.pitch_rate,ctrl_state.yaw_rate
  Flags : Subsystem
  Gain : Gain  Gain=1000000
  Parameter initialization : Subsystem
  Unit Delay : UnitDelay  SampleTime=MC_SAMPLING_PERIOD
  mc_att_control_main : MATLAB Function  TreatAsAtomicUnit=on  SystemSampleTime=MC_SAMPLING_PERIOD
  actuatorsControl : Outport  SampleTime=MC_SAMPLING_PERIOD
  bus : Outport  Port=2  SampleTime=MC_SAMPLING_PERIOD
  wires:
  flags/1 -> Demux1/1
  nuBody/1 -> Demux/1
  q/1 -> Feedback inputs/2
  armed/1 -> Flags/1(armed)
  Demux1/1 -> Flags/2(control_attitude)
  Demux1/2 -> Flags/3(control_auto)
  Demux1/3 -> Flags/4(control_manual)
  Demux1/4 -> Flags/5(control_rates)
  Demux1/5 -> Flags/6(control_velocity)
  yawRateDes/1 -> Control inputs/4
  thrustDes/1 -> Control inputs/3
  qDes/1 -> Control inputs/2
  Feedback inputs/1 -> Control inputs/1
  Gain/1 -> mc_att_control_main/1(hrt_absolute_time)
  Clock/1 -> Gain/1
  Demux/3 -> Feedback inputs/5
  Demux/2 -> Feedback inputs/4
  Demux/1 -> Feedback inputs/3
  Flags/1(Bus) -> Feedback inputs/1
  Control inputs/1 -> mc_att_control_main/3(self)
  Unit Delay/1 -> Flags/7(BusIn)
  Bus Selector1/1 -> actuatorsControl/1  "<control>"
  Parameter initialization/1(parameters) -> mc_att_control_main/2(parameters)
  mc_att_control_main/1(selfOut) -> Bus Selector1/1, Unit Delay/1, bus/1

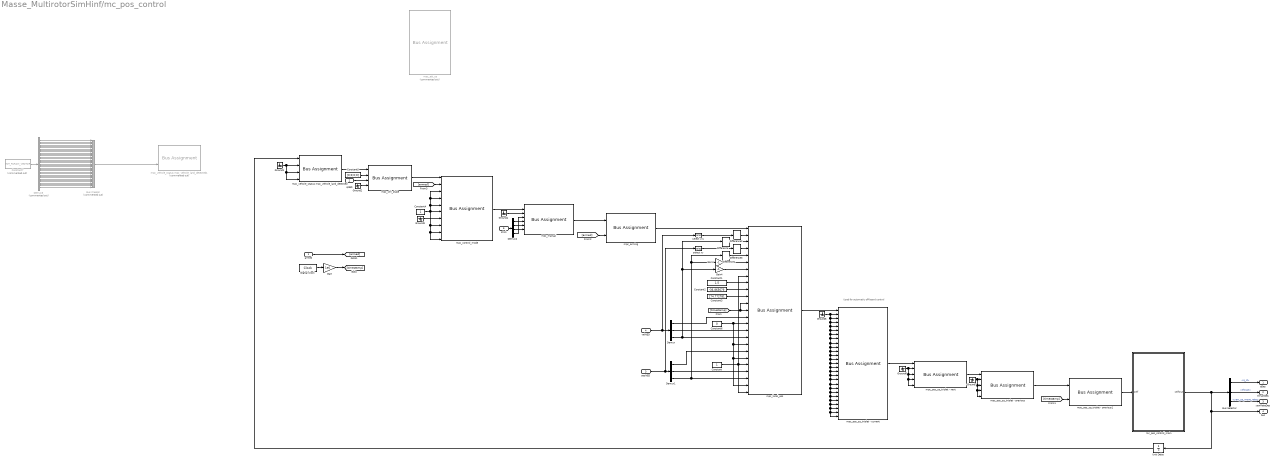
== system Masse_MultirotorSimHinf/mc_pos_control ==
  note: Used for automatic off-board control
  armed : Inport  PortDimensions=1  SampleTime=MPC_SAMPLING_PERIOD
  qNED : Inport  Port=2  PortDimensions=4  SampleTime=MPC_SAMPLING_PERIOD
  posNED : Inport  Port=3  PortDimensions=3  SampleTime=MPC_SAMPLING_PERIOD
  velNED : Inport  Port=4  PortDimensions=3  SampleTime=MPC_SAMPLING_PERIOD
  stick : Inport  Port=5  PortDimensions=4  SampleTime=MPC_SAMPLING_PERIOD
  Bus Creator : BusCreator  Commented=on  Inputs=35  OutDataTypeStr=Bus: mpc_param_find
  Bus Selector : BusSelector  OutputSignals=mpc_att_sp.q_d,mpc_att_sp.thrust,mpc_att_sp.yaw_sp_move_rate
  Constant : Constant  SampleTime=MPC_SAMPLING_PERIOD
  Constant1 : Constant  Value=1.5  SampleTime=MPC_SAMPLING_PERIOD
  Constant2 : Constant  Value=-36.865679  SampleTime=MPC_SAMPLING_PERIOD
  Constant3 : Constant  Value=174.772781  SampleTime=MPC_SAMPLING_PERIOD
  Constant4 : Constant
  Constant5 : Constant  Value=[0;0;0;0]
  Constant6 : Constant  Value=0  SampleTime=MPC_SAMPLING_PERIOD
  Constant7 : Constant  Commented=on  Value=INIT_PARAM_VECTOR
  Demux : Demux  Outputs=3
  Demux1 : Demux  Outputs=3
  Demux2 : Demux
  Demux3 : Demux  Commented=on  Outputs=35
  Difference{,1..3} (4 alike) : simulink/Discrete/Difference  ICPrevInput=0.0  OutMin=[]  OutMax=[]  OutDataType=fixdt(1, 16)  OutScaling=2^-10  DoSatur=off
  Digital Clock : DigitalClock  SampleTime=MPC_SAMPLING_PERIOD
  Gain : Gain  Gain=1e6
  Gain1 : Gain  Gain=-1
  Gain4 : Gain  Gain=-1
  Ground{1..7} (7 alike) : Ground
  Unit Delay : UnitDelay  InitialCondition=MPC_INIT_SELF  SampleTime=MPC_SAMPLING_PERIOD
  mc_pos_control_main : MATLAB Function  TreatAsAtomicUnit=on  SystemSampleTime=MPC_SAMPLING_PERIOD
  mpc_arming : BusAssignment  AssignedSignals=mpc_arming.armed
  mpc_att_sp : BusAssignment  Commented=on  AssignedSignals=mpc_att_sp.disable_mc_yaw_control,mpc_att_sp.landing_gear,mpc_att_sp.pitch_body,mpc_att_sp.q_d,mpc_att_sp.q_d_valid,mpc_att_sp.roll_body,mpc_att_sp.thrust,mpc_att_sp.timestamp,mpc_att_sp.yaw_body,mpc_att_sp.yaw_sp_move_rate
  mpc_control_mode : BusAssignment  AssignedSignals=mpc_control_mode.flag_armed,mpc_control_mode.flag_control_acceleration_enabled,mpc_control_mode.flag_control_altitude_enabled,mpc_control_mode.flag_control_climb_rate_enabled,mpc_control_mode.flag_control_manual_enabled,mpc_control_mode.flag_control_offboard_enabled,mpc_control_mode.flag_control_position_enabled,mpc_control_mode.flag_control_velocity_enabled,mpc_control_mode.flag_control_attitude_enabled
  mpc_ctrl_state : BusAssignment  AssignedSignals=mpc_ctrl_state.delta_q_reset,mpc_ctrl_state.q,mpc_ctrl_state.quat_reset_counter
  mpc_local_pos : BusAssignment  AssignedSignals=mpc_local_pos.delta_vxy,mpc_local_pos.delta_vz,mpc_local_pos.delta_xy,mpc_local_pos.delta_z,mpc_local_pos.dist_bottom,mpc_local_pos.dist_bottom_rate,mpc_local_pos.dist_bottom_valid,mpc_local_pos.ref_alt,mpc_local_pos.ref_lat,mpc_local_pos.ref_lon,mpc_local_pos.ref_timestamp,mpc_local_pos.timestamp,mpc_local_pos.vx,mpc_local_pos.vxy_reset_counter,mpc_local_pos.vy,mpc_local_pos.vz,mpc_local_pos.vz_reset_counter,mpc_local_pos.x,mpc_local_pos.xy_reset_counter,mpc_local_pos.xy_valid,mpc_local_pos.y,mpc_local_pos.z,mpc_local_pos.z_reset_counter,mpc_local_pos.z_valid
  mpc_manual : BusAssignment  AssignedSignals=mpc_manual.gear_switch,mpc_manual.r,mpc_manual.x,mpc_manual.y,mpc_manual.z
  mpc_pos_sp_triplet - current : BusAssignment  AssignedSignals=mpc_pos_sp_triplet.mpc_current.a_x,mpc_pos_sp_triplet.mpc_current.a_y,mpc_pos_sp_triplet.mpc_current.a_z,mpc_pos_sp_triplet.mpc_current.acceleration_valid,mpc_pos_sp_triplet.mpc_current.acceptance_radius,mpc_pos_sp_triplet.mpc_current.alt,mpc_pos_sp_triplet.mpc_current.alt_valid,mpc_pos_sp_triplet.mpc_current.cruising_speed,mpc_pos_sp_triplet.mpc_current.disable_mc_yaw_control,mpc_pos_sp_triplet.mpc_current.lat,mpc_pos_sp_triplet.mpc_current.lon,mpc_pos_sp_triplet.mpc_current.position_valid,mpc_pos_sp_triplet.mpc_current.type,mpc_pos_sp_triplet.mpc_current.valid,mpc_pos_sp_triplet.mpc_current.velocity_frame,mpc_pos_sp_triplet.mpc_current.velocity_valid,mpc_pos_sp_triplet.mpc_current.vx,mpc_pos_sp_triplet.mpc_current.vy,mpc_pos_sp_triplet.mpc_current.vz,mpc_pos_sp_triplet.mpc_current.x,mpc_pos_sp_triplet.mpc_current.y,mpc_pos_sp_triplet.mpc_current.yaw,mpc_pos_sp_triplet.mpc_current.yaw_valid,mpc_pos_sp_triplet.mpc_current.yawspeed,mpc_pos_sp_triplet.mpc_current.yawspeed_valid,mpc_pos_sp_triplet.mpc_current.z
  mpc_pos_sp_triplet - next : BusAssignment  AssignedSignals=mpc_pos_sp_triplet.mpc_next.alt,mpc_pos_sp_triplet.mpc_next.lat,mpc_pos_sp_triplet.mpc_next.lon,mpc_pos_sp_triplet.mpc_next.valid
  mpc_pos_sp_triplet - previous : BusAssignment  AssignedSignals=mpc_pos_sp_triplet.mpc_previous.alt,mpc_pos_sp_triplet.mpc_previous.lat,mpc_pos_sp_triplet.mpc_previous.lon,mpc_pos_sp_triplet.mpc_previous.valid
  mpc_pos_sp_triplet - previous1 : BusAssignment  AssignedSignals=mpc_hrt_absolute_time
  mpc_vehicle_status mpc_vehicle_land_detected : BusAssignment  AssignedSignals=mpc_vehicle_status.is_rotary_wing,mpc_vehicle_status.is_vtol,mpc_vehicle_land_detected.landed
  mpc_vehicle_status mpc_vehicle_land_detected1 : BusAssignment  Commented=on  AssignedSignals=mpc_param_find
  select vxy : Selector  InputPortWidth=3  IndexOptions=Index vector (dialog)  Indices=[1 2]  OutputSizes=1
  select xy : Selector  InputPortWidth=3  IndexOptions=Index vector (dialog)  Indices=[1 2]  OutputSizes=1
  qDes : Outport  PortDimensions=4  SampleTime=MPC_SAMPLING_PERIOD
  thrustDes : Outport  Port=2  PortDimensions=1  SampleTime=MPC_SAMPLING_PERIOD
  yawRateDes : Outport  Port=3  PortDimensions=1  SampleTime=MPC_SAMPLING_PERIOD
  bus : Outport  Port=4  SampleTime=MPC_SAMPLING_PERIOD
  wires:
  Bus Selector/1 -> qDes/1  "<q_d>"
  Bus Selector/2 -> thrustDes/1  "<thrust>"
  Bus Selector/3 -> yawRateDes/1  "<yaw_sp_move_rate>"
  Gain1/1 -> mpc_local_pos/6
  Demux1/3 -> Difference1/1, Gain1/1, mpc_local_pos/23
  Demux3/35 -> Bus Creator/35
  Constant7/1 -> Demux3/1
  Demux3/34 -> Bus Creator/34
  Demux3/33 -> Bus Creator/33
  Demux3/32 -> Bus Creator/32
  Demux3/31 -> Bus Creator/31
  Demux3/30 -> Bus Creator/30
  Demux3/29 -> Bus Creator/29
  Demux3/28 -> Bus Creator/28
  Demux3/27 -> Bus Creator/27
  Demux3/26 -> Bus Creator/26
  Demux3/25 -> Bus Creator/25
  Demux3/24 -> Bus Creator/24
  Demux3/23 -> Bus Creator/23
  Demux3/22 -> Bus Creator/22
  Demux3/21 -> Bus Creator/21
  Demux3/20 -> Bus Creator/20
  Demux3/19 -> Bus Creator/19
  Demux3/18 -> Bus Creator/18
  Demux3/17 -> Bus Creator/17
  Demux3/16 -> Bus Creator/16
  Demux3/15 -> Bus Creator/15
  Demux3/14 -> Bus Creator/14
  Demux3/13 -> Bus Creator/13
  Demux3/12 -> Bus Creator/12
  Demux3/11 -> Bus Creator/11
  Demux3/10 -> Bus Creator/10
  Demux3/9 -> Bus Creator/9
  Demux3/8 -> Bus Creator/8
  Demux3/7 -> Bus Creator/7
  Demux3/6 -> Bus Creator/6
  Demux3/5 -> Bus Creator/5
  Demux3/4 -> Bus Creator/4
  Demux3/3 -> Bus Creator/3
  Demux3/2 -> Bus Creator/2
  Demux3/1 -> Bus Creator/1
  Bus Creator/1 -> mpc_vehicle_status mpc_vehicle_land_detected1/2
  Unit Delay/1 -> mpc_vehicle_status mpc_vehicle_land_detected/1
  Constant5/1 -> mpc_ctrl_state/2
  Demux/3 -> Gain4/1, Difference/1, mpc_local_pos/17
  [armed] -> mpc_control_mode/2
  [armed] -> mpc_arming/2
  armed/1 -> [armed]
  Ground7/1 -> mpc_pos_sp_triplet - previous/2, mpc_pos_sp_triplet - previous/3, mpc_pos_sp_triplet - previous/4, mpc_pos_sp_triplet - previous/5
  Ground6/1 -> mpc_pos_sp_triplet - next/2, mpc_pos_sp_triplet - next/3, mpc_pos_sp_triplet - next/4, mpc_pos_sp_triplet - next/5
  Ground5/1 -> mpc_pos_sp_triplet - current/2, mpc_pos_sp_triplet - current/4, mpc_pos_sp_triplet - current/27, mpc_pos_sp_triplet - current/26, mpc_pos_sp_triplet - current/25, mpc_pos_sp_triplet - current/24, mpc_pos_sp_triplet - current/23, mpc_pos_sp_triplet - current/22, mpc_pos_sp_triplet - current/21, mpc_pos_sp_triplet - current/20, mpc_pos_sp_triplet - current/19, mpc_pos_sp_triplet - current/18, mpc_pos_sp_triplet - current/17, mpc_pos_sp_triplet - current/16, mpc_pos_sp_triplet - current/15, mpc_pos_sp_triplet - current/14, mpc_pos_sp_triplet - current/13, mpc_pos_sp_triplet - current/12, mpc_pos_sp_triplet - current/11, mpc_pos_sp_triplet - current/10, mpc_pos_sp_triplet - current/9, mpc_pos_sp_triplet - current/8, mpc_pos_sp_triplet - current/7, mpc_pos_sp_triplet - current/6, mpc_pos_sp_triplet - current/5, mpc_pos_sp_triplet - current/3
  Demux2/4 -> mpc_manual/3
  Demux2/3 -> mpc_manual/6
  Demux2/2 -> mpc_manual/5
  Demux2/1 -> mpc_manual/4
  stick/1 -> Demux2/1
  Ground4/1 -> mpc_manual/2
  Ground3/1 -> mpc_control_mode/7
  Constant4/1 -> mpc_control_mode/3, mpc_control_mode/4, mpc_control_mode/5, mpc_control_mode/9, mpc_control_mode/10, mpc_control_mode/8, mpc_control_mode/6
  Ground2/1 -> mpc_ctrl_state/4
  Ground1/1 -> mpc_vehicle_status mpc_vehicle_land_detected/2, mpc_vehicle_status mpc_vehicle_land_detected/3, mpc_vehicle_status mpc_vehicle_land_detected/4
  select xy/1 -> Difference3/1
  Difference3/1 -> mpc_local_pos/4
  select vxy/1 -> Difference2/1
  Difference2/1 -> mpc_local_pos/2
  Difference/1 -> mpc_local_pos/3
  Difference1/1 -> mpc_local_pos/5
  Gain4/1 -> mpc_local_pos/7
  Demux1/2 -> mpc_local_pos/22
  Demux1/1 -> mpc_local_pos/19
  posNED/1 -> Demux1/1, select xy/1
  Demux/1 -> mpc_local_pos/14
  Demux/2 -> mpc_local_pos/16
  velNED/1 -> select vxy/1, Demux/1
  Constant2/1 -> mpc_local_pos/10
  Constant3/1 -> mpc_local_pos/11
  Constant1/1 -> mpc_local_pos/9
  [timestamp] -> mpc_pos_sp_triplet - previous1/2
  mpc_pos_sp_triplet - previous1/1 -> mc_pos_control_main/1(self)
  [timestamp] -> mpc_local_pos/13, mpc_local_pos/12
  Gain/1 -> [timestamp]
  Digital Clock/1 -> Gain/1
  Constant/1 -> mpc_local_pos/21, mpc_local_pos/8, mpc_local_pos/25
  Constant6/1 -> mpc_local_pos/15, mpc_local_pos/18, mpc_local_pos/20, mpc_local_pos/24
  mpc_pos_sp_triplet - previous/1 -> mpc_pos_sp_triplet - previous1/1
  mpc_pos_sp_triplet - next/1 -> mpc_pos_sp_triplet - previous/1
  mpc_pos_sp_triplet - current/1 -> mpc_pos_sp_triplet - next/1
  mpc_local_pos/1 -> mpc_pos_sp_triplet - current/1
  mpc_arming/1 -> mpc_local_pos/1
  mpc_manual/1 -> mpc_arming/1
  mpc_ctrl_state/1 -> mpc_control_mode/1
  mpc_control_mode/1 -> mpc_manual/1
  mpc_vehicle_status mpc_vehicle_land_detected/1 -> mpc_ctrl_state/1
  qNED/1 -> mpc_ctrl_state/3
  mc_pos_control_main/1(selfOut) -> Bus Selector/1, bus/1, Unit Delay/1

== system Masse_MultirotorSimHinf/pos_NWUtoNED1 ==
  posNWU : Inport
  Multiply : Product  Inputs=**
  Position gain : Constant  Value=[1; -1; -1]
  posNED : Outport
  wires:
  posNWU/1 -> Multiply/1
  Multiply/1 -> posNED/1
  Position gain/1 -> Multiply/2

== system Masse_MultirotorSimHinf/pos_NWUtoNED2 ==
  posNWU : Inport
  Multiply : Product  Inputs=**
  Position gain : Constant  Value=[1; -1; -1]
  posNED : Outport
  wires:
  posNWU/1 -> Multiply/1
  Multiply/1 -> posNED/1
  Position gain/1 -> Multiply/2

== system Masse_MultirotorSimHinf/pos_q_NWUtoNED ==
  qNWU : Inport
  Multiply : Product  Inputs=**
  Quaternion gain : Constant  Value=[1; 1; -1; -1]
  qNED : Outport
  wires:
  Quaternion gain/1 -> Multiply/2
  Multiply/1 -> qNED/1
  qNWU/1 -> Multiply/1

== system Masse_MultirotorSimHinf/Applied wind speed/Quaternion to Rotation Matrix1 ==
  quaternion : Inport
  MATLAB Function : MATLAB Function  TreatAsAtomicUnit=on
  rotationMatrix : Outport
  wires:
  MATLAB Function/1(R) -> rotationMatrix/1
  quaternion/1 -> MATLAB Function/1(q)

== system Masse_MultirotorSimHinf/Quadrotor Euler Model/Euler Angles to Quaternion ==
  euler : Inport
  MATLAB Function : MATLAB Function  TreatAsAtomicUnit=on
  quaternion : Outport
  wires:
  MATLAB Function/1(quat) -> quaternion/1
  euler/1 -> MATLAB Function/1(eulerAngles)

== system Masse_MultirotorSimHinf/Quadrotor Quaternion Model/Compute S Matrix1 ==
  quaternion : Inport
  MATLAB Function : MATLAB Function  TreatAsAtomicUnit=on
  rotationMatrix : Outport
  wires:
  quaternion/1 -> MATLAB Function/1(q)
  MATLAB Function/1(S) -> rotationMatrix/1
